simulink model "RobotLocalisation_no_external_mode"  (R2013b)
settings: Solver=FixedStepDiscrete  StartTime=0.0  StopTime=inf  FixedStep=1/30  RelTol=1e-3
PreLoadFcn:
  | force_config
PostLoadFcn:
  | load_scoring_params
values from neighbouring files (symbols this model uses):
  allotedRunTime = 3*60    (= 180)    [load_scoring_params.m]
  startingRadius = 0.1    [load_scoring_params.m]
  startPos = [0.5, 0.5]    [load_scoring_params.m]
  statTimeReq = 2.5    [load_scoring_params.m]
  targetBoundaryRadius = 0.07    [load_scoring_params.m]
undefined symbols (not defined in the file or in its folder): Green, led0, magnitude
libraries: simulink x9, embdlinuxlib x6, visionstatistics x2, visiongeotforms x1
settings Model: ExtModeTrigDuration=100  Creator=omcaree  LastModifiedBy=radams
settings OptimizationCC: InlineParams=on  UseFloatMulNetSlope=on  UseSpecifiedMinMax=on  InlineInvariantSignals=on  EnhancedBackFolding=on  BooleansAsBitfields=on  PassReuseOutputArgsAs=Individual arguments  StateBitsets=on  DataBitsets=on  ZeroExternalMemoryAtStartup=off  ZeroInternalMemoryAtStartup=off  EfficientFloat2IntCast=on  OptimizeModelRefInitCode=on  LifeSpan=1
settings DebuggingCC: SolverPrmCheckMsg=none
settings HardwareCC: ProdLargestAtomicInteger=Long  ProdLargestAtomicFloat=Double  ProdEndianess=LittleEndian  ProdHWDeviceType=ARM Compatible->ARM Cortex
settings RTWCC: SystemTargetFile=realtime.tlc  GenerateMakefile=off  TemplateMakefile=realtime.tmf  Description=Run on Target Hardware  RTWVerbose=off  ProcessScript=realtime_make_rtw_hook  CustomSourceCode="#include \"send_udp.h\""  CustomSource=send_udp.c  IncludeHyperlinkInReport=on  RTWCompilerOptimization=On
settings STFCustomTargetCC: TargetLibSuffix=.a  GenerateSampleERTMain=on  CombineSignalStateStructs=on  SuppressErrorStatus=on  ERTCustomFileBanners=on  SupportNonInlinedSFcns=off  SupportVariableSizeSignals=on  MATLABClassNameForMDSCustomization=Simulink.SoftwareTarget.ERTCustomization  GRTInterface=off  SystemTargetFile=realtime.tlc
settings ERTTargetCC: CodeReplacementLibrary=ANSI_C  GenerateSampleERTMain=on  ParMdlRefBuildCompliant=off  CompOptLevelCompliant=off  ConcurrentExecutionCompliant=off  CombineOutputUpdateFcns=off  CombineSignalStateStructs=on  SuppressErrorStatus=on  ERTFirstTimeCompliant=off  SupportContinuousTime=on  SupportVariableSizeSignals=on  ModelStepFunctionPrototypeControlCompliant=off  CPPClassGenCompliant=off  ExtModeMexArgs='169.254.0.30' 0 17725  InlinedParameterPlacement=NonHierarchical  ERTSrcFileBannerTemplate=realtime_code_template.cgt  ERTHdrFileBannerTemplate=realtime_code_template.cgt  ERTDataSrcFileTemplate=realtime_code_template.cgt  ERTDataHdrFileTemplate=realtime_code_template.cgt  ERTCustomFileTemplate=realtime_file_process.tlc  ConvertIfToSwitch=on  SuppressUnreachableDefaultCases=on

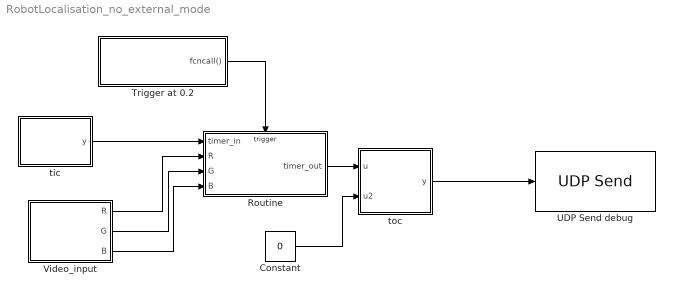
== system RobotLocalisation_no_external_mode ==
  Constant : Constant  Value=0
  Routine : Subsystem  TreatAsAtomicUnit=on
  Trigger at 0.2 : MATLAB Function  TreatAsAtomicUnit=on
  UDP Send debug : embdlinuxlib/UDP Send  remoteURL='169.254.230.213'  remotePort=17728  localURL='255.255.255.255'  localPortSource=Automatically determine  localPort=-1  sampletime=-1  blockPlatform=Raspberry Pi  separateLengthPort=0
  Video_input : Subsystem  TreatAsAtomicUnit=on
  tic : MATLAB Function  TreatAsAtomicUnit=on
  toc : MATLAB Function  TreatAsAtomicUnit=on
  wires:
  Routine/1(timer_out) -> toc/1(u)
  toc/1(y) -> UDP Send debug/1
  tic/1(y) -> Routine/1(timer_in)
  Video_input/1(R) -> Routine/2(R)
  Video_input/2(G) -> Routine/3(G)
  Video_input/3(B) -> Routine/4(B)
  Trigger at 0.2/1(fcncall()) -> Routine/Trigger
  Constant/1 -> toc/2(u2)

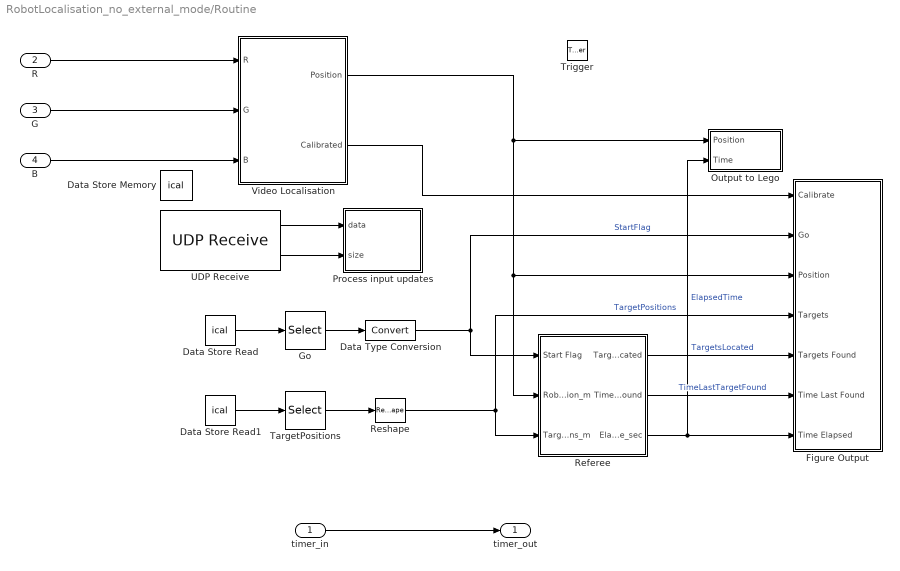
== system RobotLocalisation_no_external_mode/Routine ==
  timer_in : Inport
  R : Inport  Port=2
  G : Inport  Port=3
  B : Inport  Port=4
  Trigger : TriggerPort  TriggerType=function-call  PortDimensions=1
  Data Store Memory : DataStoreMemory  DataStoreName=ical  ReadBeforeWriteMsg=warning  WriteAfterWriteMsg=warning  WriteAfterReadMsg=warning  InitialValue=zeros(22,1)  OutDataTypeStr=double
  Data Store Read : DataStoreRead  DataStoreName=ical
  Data Store Read1 : DataStoreRead  DataStoreName=ical
  Data Type Conversion : DataTypeConversion
  Figure Output : Subsystem
  Go : Selector  InputPortWidth=22  IndexOptions=Index vector (dialog)  Indices=1  OutputSizes=1
  Output to Lego : Subsystem
  Process input updates : MATLAB Function  TreatAsAtomicUnit=on
  Referee : Subsystem
      mask Display: image(imread('referee.png'))
  Reshape : Reshape  OutputDimensionality=Customize  OutputDimensions=[9 2]
  TargetPositions : Selector  InputPortWidth=22  IndexOptions=Index vector (dialog)  Indices=[2:19]  OutputSizes=1
  UDP Receive : embdlinuxlib/UDP Receive  localURL='0.0.0.0'  localPort=17727  remoteURL='0.0.0.0'  remotePort=-1  recvBufferSize=8192  signalDatatype=uint8  dims=176  isVarSize=off  showBlockingTime=off  blockingTime=0  sampletime=-1  blockPlatform=Raspberry Pi
  Video Localisation : Subsystem
  timer_out : Outport
  wires:
  Data Type Conversion/1 -> Referee/1(Start Flag), Figure Output/2(Go)  "StartFlag"
  Referee/1(Targets Located) -> Figure Output/5(Targets Found)  "TargetsLocated"
  Reshape/1 -> Referee/3(Target Positions_m), Figure Output/4(Targets)  "TargetPositions"
  Video Localisation/1(Position) -> Referee/2(Robot Position_m), Figure Output/3(Position), Output to Lego/1(Position)
  Video Localisation/2(Calibrated) -> Figure Output/1(Calibrate)
  Referee/2(Time Last Target Found) -> Figure Output/6(Time Last Found)  "TimeLastTargetFound"
  Referee/3(Elapsed Time_sec) -> Output to Lego/2(Time), Figure Output/7(Time Elapsed)  "ElapsedTime"
  UDP Receive/1 -> Process input updates/1(data)
  UDP Receive/2 -> Process input updates/2(size)
  Data Store Read/1 -> Go/1
  Go/1 -> Data Type Conversion/1
  TargetPositions/1 -> Reshape/1
  Data Store Read1/1 -> TargetPositions/1
  timer_in/1 -> timer_out/1
  R/1 -> Video Localisation/1(R)
  G/1 -> Video Localisation/2(G)
  B/1 -> Video Localisation/3(B)

== system RobotLocalisation_no_external_mode/Video_input ==
  V4L2 Video Capture : embdlinuxlib/V4L2 Video Capture  m_devName='/dev/video0'  roi=[0, 0, 640, 480]  imSizeSelection=320x240  imSize=[640, 480]  pixelFormat=RGB  pixelOrder=Planar  sampleTime=1/30  simOutput=Colorbars  blockPlatform=Raspberry Pi
  R : Outport
  G : Outport  Port=2
  B : Outport  Port=3
  wires:
  V4L2 Video Capture/3 -> B/1
  V4L2 Video Capture/2 -> G/1
  V4L2 Video Capture/1 -> R/1

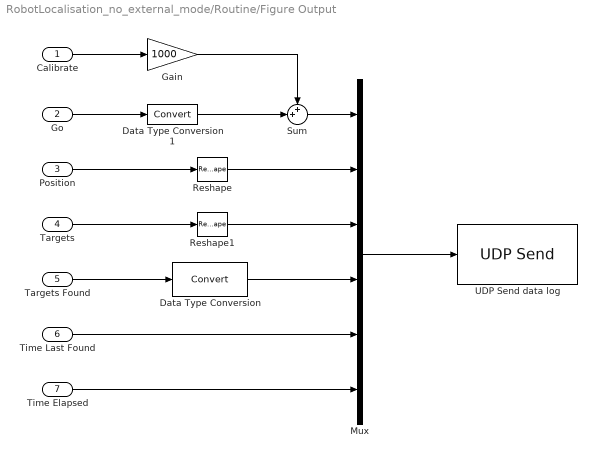
== system RobotLocalisation_no_external_mode/Routine/Figure Output ==
  Calibrate : Inport
  Go : Inport  Port=2
  Position : Inport  Port=3
  Targets : Inport  Port=4
  Targets Found : Inport  Port=5
  Time Last Found : Inport  Port=6
  Time Elapsed : Inport  Port=7
  Data Type Conversion : DataTypeConversion
  Data Type Conversion1 : DataTypeConversion
  Gain : Gain  Gain=1000  OutDataTypeStr=double
  Mux : Mux  Inputs=6
  Reshape : Reshape
  Reshape1 : Reshape
  Sum : Sum  Inputs=++|
  UDP Send data log : embdlinuxlib/UDP Send  remoteURL='169.254.230.213'  remotePort=17726  localURL='255.255.255.255'  localPortSource=Automatically determine  localPort=-1  sampletime=-1  blockPlatform=Raspberry Pi  separateLengthPort=0
  wires:
  Targets/1 -> Reshape1/1
  Targets Found/1 -> Data Type Conversion/1
  Time Last Found/1 -> Mux/5
  Time Elapsed/1 -> Mux/6
  Mux/1 -> UDP Send data log/1
  Position/1 -> Reshape/1
  Data Type Conversion/1 -> Mux/4
  Reshape/1 -> Mux/2
  Reshape1/1 -> Mux/3
  Calibrate/1 -> Gain/1
  Sum/1 -> Mux/1
  Go/1 -> Data Type Conversion1/1
  Gain/1 -> Sum/1
  Data Type Conversion1/1 -> Sum/2

== system RobotLocalisation_no_external_mode/Routine/Output to Lego ==
  Position : Inport
  Time : Inport  Port=2
  Data Type Conversion1 : DataTypeConversion  OutDataTypeStr=int32
  Demux1 : Demux  Outputs=2
  Gain3 : Gain  Gain=10  ParamDataTypeStr=uint8
  Gain4 : Gain  Gain=100  ParamDataTypeStr=uint8
  Gain5 : Gain  Gain=100  ParamDataTypeStr=uint8
  Mux1 : Mux  Inputs=3
  UDP Send2 : embdlinuxlib/UDP Send  remoteURL='127.0.0.1'  remotePort=32000  localURL='255.255.255.255'  localPortSource=Automatically determine  localPort=-1  sampletime=-1  blockPlatform=Raspberry Pi  separateLengthPort=0
  wires:
  Position/1 -> Demux1/1
  Time/1 -> Gain3/1
  Mux1/1 -> Data Type Conversion1/1
  Data Type Conversion1/1 -> UDP Send2/1
  Demux1/1 -> Gain4/1
  Demux1/2 -> Gain5/1
  Gain4/1 -> Mux1/2
  Gain5/1 -> Mux1/3
  Gain3/1 -> Mux1/1

== system RobotLocalisation_no_external_mode/Routine/Referee ==
  Start Flag : Inport  OutDataTypeStr=boolean
  Robot Position_m : Inport  Port=2
  Target Positions_m : Inport  Port=3
  Chart (MATLAB) : Stateflow chart  TreatAsAtomicUnit=on
  Reshape : Reshape  OutputDimensionality=Row vector (2-D)
  Targets Located : Outport
  Time Last Target Found : Outport  Port=2  PortDimensions=1
  Elapsed Time_sec : Outport  Port=3  PortDimensions=1
  wires:
  Chart (MATLAB)/1(timeLastTargetFound) -> Time Last Target Found/1
  Chart (MATLAB)/3(targetsFound) -> Targets Located/1
  Robot Position_m/1 -> Reshape/1
  Start Flag/1 -> Chart (MATLAB)/2(StartFlag)
  Reshape/1 -> Chart (MATLAB)/1(robotPosition)
  Target Positions_m/1 -> Chart (MATLAB)/3(targetPositions)
  Chart (MATLAB)/2(elapsedTime) -> Elapsed Time_sec/1

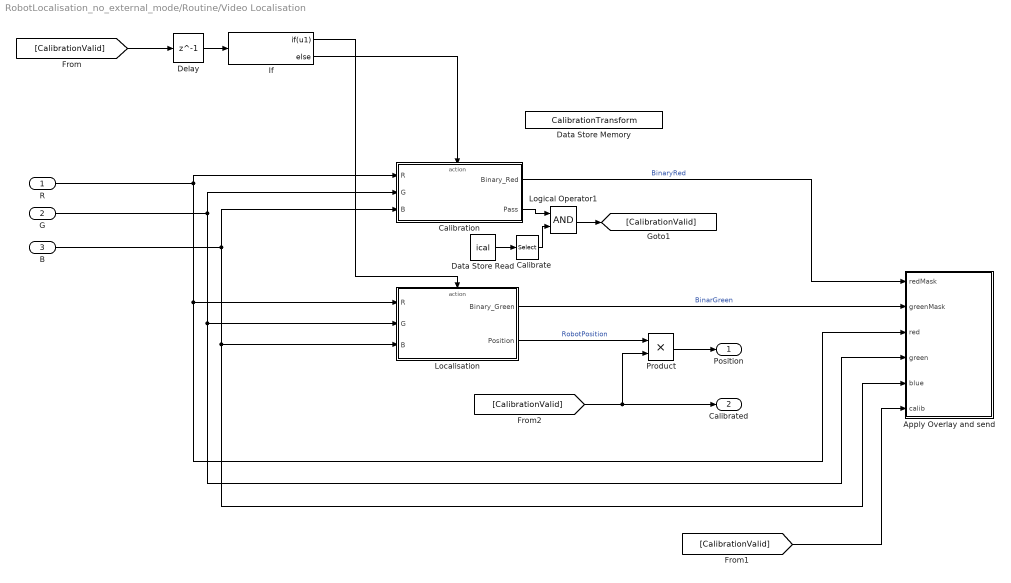
== system RobotLocalisation_no_external_mode/Routine/Video Localisation ==
  R : Inport
  G : Inport  Port=2
  B : Inport  Port=3
  Apply Overlay and send : MATLAB Function
  Calibrate : Selector  InputPortWidth=22  IndexOptions=Index vector (dialog)  Indices=22  OutputSizes=1
  Calibration : Subsystem  TreatAsAtomicUnit=on
      settings: RTWSystemCode=Inline
  Data Store Memory : DataStoreMemory  DataStoreName=CalibrationTransform  ReadBeforeWriteMsg=warning  WriteAfterWriteMsg=warning  WriteAfterReadMsg=warning  InitialValue=[1 0 0; 0 1 0; 0 0 1]  VectorParams1D=off  Dimensions=[3 3]
  Data Store Read : DataStoreRead  DataStoreName=ical
  Delay : Delay  DelayLength=1  InitialCondition=0
  If : If  IfExpression=u1
  Localisation : Subsystem  TreatAsAtomicUnit=on
      settings: RTWSystemCode=Inline
  Logical Operator1 : Logic  AllPortsSameDT=off  OutDataTypeStr=boolean
  Product : Product  OutDataTypeStr=double
  Position : Outport
  Calibrated : Outport  Port=2
  wires:
  Delay/1 -> If/1
  [CalibrationValid] -> Delay/1
  Localisation/2(Position) -> Product/1  "RobotPosition"
  Product/1 -> Position/1
  Data Store Read/1 -> Calibrate/1
  Calibration/2(Pass) -> Logical Operator1/1
  Calibrate/1 -> Logical Operator1/2
  Logical Operator1/1 -> [CalibrationValid]
  [CalibrationValid] -> Product/2, Calibrated/1
  Calibration/1(Binary_Red) -> Apply Overlay and send/1(redMask)  "BinaryRed"
  Localisation/1(Binary_Green) -> Apply Overlay and send/2(greenMask)  "BinarGreen"
  R/1 -> Calibration/1(R), Apply Overlay and send/3(red), Localisation/1(R)
  G/1 -> Apply Overlay and send/4(green), Localisation/2(G), Calibration/2(G)
  B/1 -> Calibration/3(B), Apply Overlay and send/5(blue), Localisation/3(B)
  If/2 -> Calibration/Action
  If/1 -> Localisation/Action
  [CalibrationValid] -> Apply Overlay and send/6(calib)

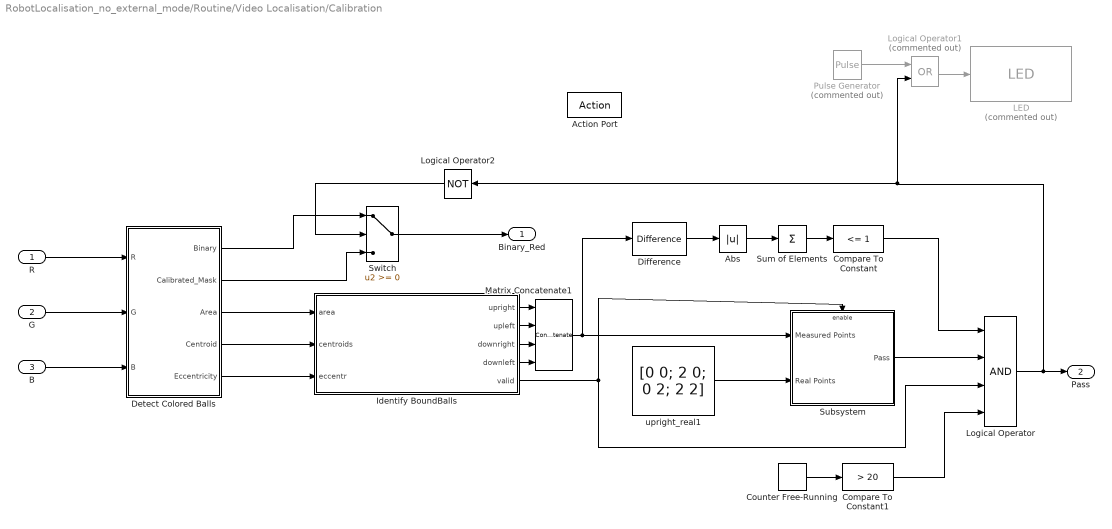
== system RobotLocalisation_no_external_mode/Routine/Video Localisation/Calibration ==
  R : Inport
  G : Inport  Port=2
  B : Inport  Port=3
  Action Port : ActionPort  ActionType=else
  Abs : Abs
  Compare To Constant : simulink/Logic and Bit Operations/Compare To Constant  relop=<=  const=1  OutDataTypeStr=boolean
  Compare To Constant1 : simulink/Logic and Bit Operations/Compare To Constant  relop=>  const=20  OutDataTypeStr=boolean
  Counter Free-Running : simulink/Sources/Counter Free-Running  NumBits=16  tsamp=-1
  Detect Colored Balls : Subsystem
  Difference : simulink/Discrete/Difference  ICPrevInput=0.0  InputProcessing=Inherited  OutMin=[]  OutMax=[]  OutDataType=fixdt(1, 16)  OutScaling=2^-10  DoSatur=off
  Identify BoundBalls : MATLAB Function  TreatAsAtomicUnit=on
  LED : embdlinuxlib/LED  Commented=on  board=Model B Rev2  led=led0 (Green)  blockPlatform=Raspberry Pi
  Logical Operator : Logic  Inputs=4  AllPortsSameDT=off  OutDataTypeStr=boolean
  Logical Operator1 : Logic  Commented=on  Operator=OR  AllPortsSameDT=off  OutDataTypeStr=boolean
  Logical Operator2 : Logic  Operator=NOT  AllPortsSameDT=off  OutDataTypeStr=boolean
  Matrix Concatenate1 : Concatenate  NumInputs=4  Mode=Multidimensional array
  Pulse Generator : DiscretePulseGenerator  Commented=on  PulseType=Time based  Period=0.4  PulseWidth=50
  Subsystem : Subsystem
  Sum of Elements : Sum  Inputs=+
  Switch : Switch
  upright_real1 : Constant  Value=[0 0; 2 0; 0 2; 2 2]  VectorParams1D=off
  Binary_Red : Outport
  Pass : Outport  Port=2
  wires:
  Identify BoundBalls/2(upleft) -> Matrix Concatenate1/2
  Identify BoundBalls/3(downright) -> Matrix Concatenate1/3
  Identify BoundBalls/4(downleft) -> Matrix Concatenate1/4
  Identify BoundBalls/1(upright) -> Matrix Concatenate1/1
  Matrix Concatenate1/1 -> Difference/1, Subsystem/1(Measured Points)
  Identify BoundBalls/5(valid) -> Logical Operator/3, Subsystem/Enable
  Difference/1 -> Abs/1
  Sum of Elements/1 -> Compare To Constant/1
  Abs/1 -> Sum of Elements/1
  Compare To Constant/1 -> Logical Operator/1
  R/1 -> Detect Colored Balls/1(R)
  G/1 -> Detect Colored Balls/2(G)
  B/1 -> Detect Colored Balls/3(B)
  Detect Colored Balls/3(Area) -> Identify BoundBalls/1(area)
  Detect Colored Balls/4(Centroid) -> Identify BoundBalls/2(centroids)
  Detect Colored Balls/5(Eccentricity) -> Identify BoundBalls/3(eccentr)
  Subsystem/1(Pass) -> Logical Operator/2
  Logical Operator/1 -> Pass/1, Logical Operator1/2, Logical Operator2/1
  Pulse Generator/1 -> Logical Operator1/1
  Logical Operator1/1 -> LED/1
  Counter Free-Running/1 -> Compare To Constant1/1
  Compare To Constant1/1 -> Logical Operator/4
  upright_real1/1 -> Subsystem/2(Real Points)
  Detect Colored Balls/1(Binary) -> Switch/1
  Detect Colored Balls/2(Calibrated_Mask) -> Switch/3
  Switch/1 -> Binary_Red/1
  Logical Operator2/1 -> Switch/2

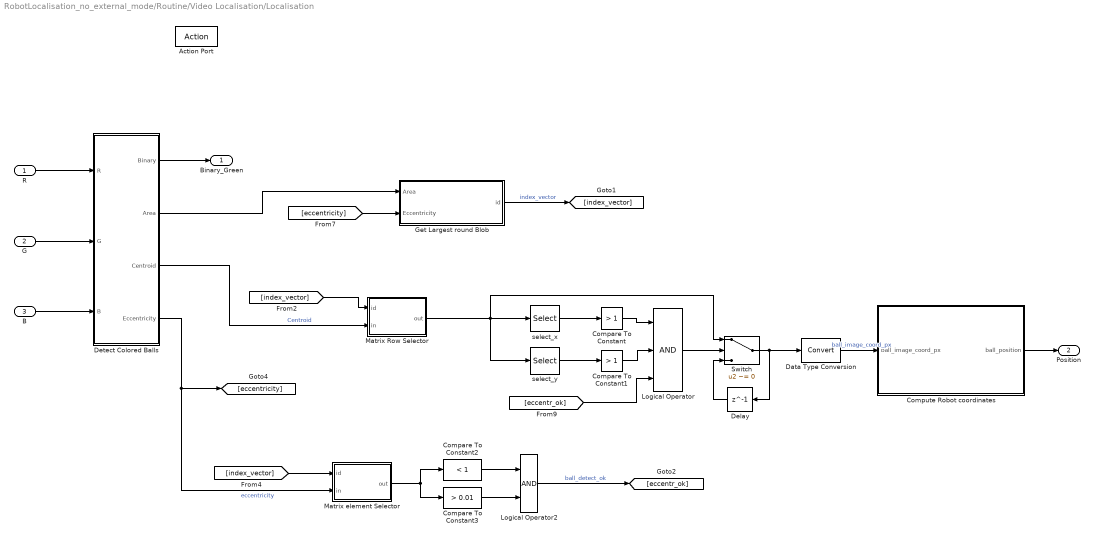
== system RobotLocalisation_no_external_mode/Routine/Video Localisation/Localisation ==
  R : Inport
  G : Inport  Port=2
  B : Inport  Port=3
  Action Port : ActionPort  ActionType=then
  Compare To Constant : simulink/Logic and Bit Operations/Compare To Constant  relop=>  const=1  OutDataTypeStr=boolean
  Compare To Constant1 : simulink/Logic and Bit Operations/Compare To Constant  relop=>  const=1  OutDataTypeStr=boolean
  Compare To Constant2 : simulink/Logic and Bit Operations/Compare To Constant  relop=<  const=1  OutDataTypeStr=boolean
  Compare To Constant3 : simulink/Logic and Bit Operations/Compare To Constant  relop=>  const=0.01  OutDataTypeStr=boolean
  Compute Robot coordinates : Subsystem
  Data Type Conversion : DataTypeConversion
  Delay : Delay  DelayLength=1  InitialCondition=320/2
  Detect Colored Balls : Subsystem
  Get Largest round Blob : MATLAB Function  TreatAsAtomicUnit=on
  Logical Operator : Logic  Inputs=3  AllPortsSameDT=off  OutDataTypeStr=boolean
  Logical Operator2 : Logic  AllPortsSameDT=off  OutDataTypeStr=boolean
  Matrix Row Selector : MATLAB Function  TreatAsAtomicUnit=on
  Matrix element Selector : MATLAB Function  TreatAsAtomicUnit=on
  Switch : Switch  Criteria=u2 ~= 0
  select_x : Selector  InputPortWidth=2  IndexOptions=Index vector (dialog)  Indices=[1 ]  OutputSizes=1
  select_y : Selector  InputPortWidth=2  IndexOptions=Index vector (dialog)  Indices=2  OutputSizes=1
  Binary_Green : Outport
  Position : Outport  Port=2
  wires:
  B/1 -> Detect Colored Balls/3(B)
  G/1 -> Detect Colored Balls/2(G)
  R/1 -> Detect Colored Balls/1(R)
  Detect Colored Balls/2(Area) -> Get Largest round Blob/1(Area)
  Switch/1 -> Data Type Conversion/1, Delay/1
  Delay/1 -> Switch/3
  select_x/1 -> Compare To Constant/1
  Compare To Constant/1 -> Logical Operator/1
  Logical Operator/1 -> Switch/2
  Get Largest round Blob/1(id) -> [index_vector]  "index_vector"
  Compare To Constant2/1 -> Logical Operator2/1
  Detect Colored Balls/4(Eccentricity) -> Matrix element Selector/2(in), [eccentricity]  "eccentricity"
  [index_vector] -> Matrix element Selector/1(id)
  Detect Colored Balls/3(Centroid) -> Matrix Row Selector/2(in)  "Centroid"
  [index_vector] -> Matrix Row Selector/1(id)
  Matrix Row Selector/1(out) -> select_y/1, select_x/1, Switch/1
  Matrix element Selector/1(out) -> Compare To Constant2/1, Compare To Constant3/1
  Compare To Constant3/1 -> Logical Operator2/2
  Logical Operator2/1 -> [eccentr_ok]  "ball_detect_ok"
  [eccentricity] -> Get Largest round Blob/2(Eccentricity)
  Data Type Conversion/1 -> Compute Robot coordinates/1(ball_image_coord_px)  "ball_image_coord_px"
  select_y/1 -> Compare To Constant1/1
  Compare To Constant1/1 -> Logical Operator/2
  [eccentr_ok] -> Logical Operator/3
  Compute Robot coordinates/1(ball_position) -> Position/1
  Detect Colored Balls/1(Binary) -> Binary_Green/1

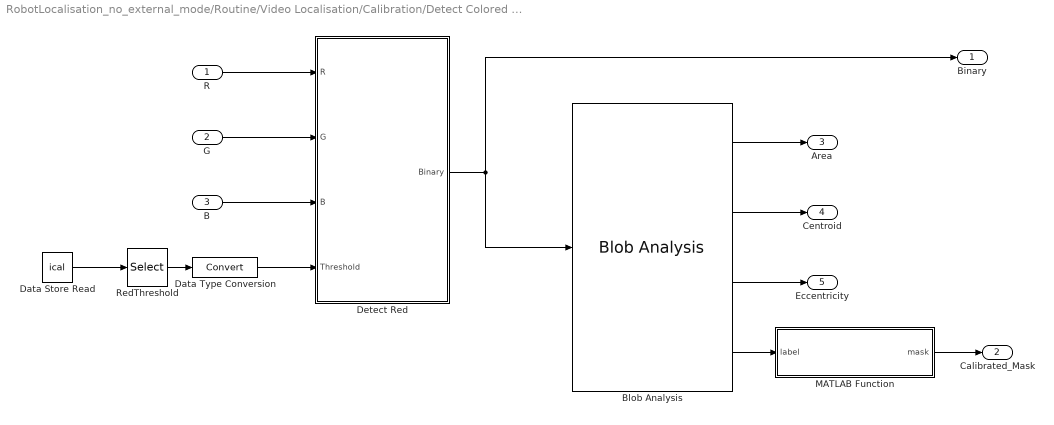
== system RobotLocalisation_no_external_mode/Routine/Video Localisation/Calibration/Detect Colored Balls ==
  R : Inport
  G : Inport  Port=2
  B : Inport  Port=3
  Blob Analysis : visionstatistics/Blob Analysis  Tag=vipblks_row_conv  area=on  centroid=on  bBox=off  majorAxis=off  minorAxis=off  angle=off  eccentricity=on  equivDiameterSq=off  extent=off  perimeter=off  maxBlobs=4  warnIfNumBlobsExceeded=on  isCount=off  useMinArea=on  minArea=10  useMaxArea=off  maxArea=15000  excludeBorderBlob=on  outDT=double  isOutVarDim=off  isFill=on  fillValues=0  conn=4  isLabel=on  outputMode=Binary point scaling  outputWordLength=32  outputFracLength=16  firstCoeffMode=Binary point scaling  firstCoeffWordLength=16  firstCoeffFracLength=14  secondCoeffMode=Binary point scaling  secondCoeffWordLength=32  secondCoeffFracLength=16  accumMode=Binary point scaling  accumWordLength=32  accumFracLength=0  prodOutputMode=Binary point scaling  prodOutputWordLength=32  prodOutputFracLength=16  roundingMode=Floor  overflowMode=off
  Data Store Read : DataStoreRead  DataStoreName=ical
  Data Type Conversion : DataTypeConversion
  Detect Red : Subsystem
  MATLAB Function : MATLAB Function  TreatAsAtomicUnit=on
  RedThreshold : Selector  InputPortWidth=22  IndexOptions=Index vector (dialog)  Indices=20  OutputSizes=1
  Binary : Outport
  Calibrated_Mask : Outport  Port=2
  Area : Outport  Port=3
  Centroid : Outport  Port=4
  Eccentricity : Outport  Port=5
  wires:
  G/1 -> Detect Red/2(G)
  R/1 -> Detect Red/1(R)
  B/1 -> Detect Red/3(B)
  Detect Red/1(Binary) -> Binary/1, Blob Analysis/1
  Blob Analysis/2 -> Centroid/1
  Blob Analysis/1 -> Area/1
  Blob Analysis/3 -> Eccentricity/1
  Data Store Read/1 -> RedThreshold/1
  RedThreshold/1 -> Data Type Conversion/1
  Data Type Conversion/1 -> Detect Red/4(Threshold)
  Blob Analysis/4 -> MATLAB Function/1(label)
  MATLAB Function/1(mask) -> Calibrated_Mask/1

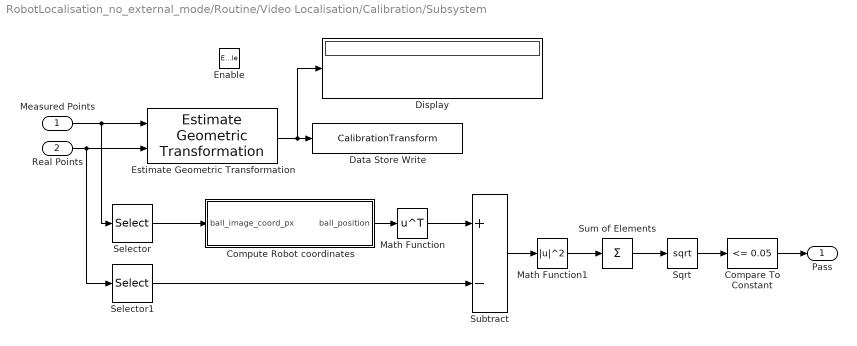
== system RobotLocalisation_no_external_mode/Routine/Video Localisation/Calibration/Subsystem ==
  Measured Points : Inport
  Real Points : Inport  Port=2
  Enable : EnablePort
  Compare To Constant : simulink/Logic and Bit Operations/Compare To Constant  relop=<=  const=0.05  OutDataTypeStr=boolean
  Compute Robot coordinates : Subsystem
  Data Store Write : DataStoreWrite  DataStoreName=CalibrationTransform
  Display : Display
  Estimate Geometric Transformation : visiongeotforms/Estimate Geometric Transformation  tformType=Projective  isRandomSampling=on  algMethod=Random Sample Consensus (RANSAC)  numMethod=Specified value  isStopSampling=off  percentStop=75  distanceAlg=2.5  distanceGeo=2.5  sampleNum=500  maxSampleNum=1000  desiredConfidence=99  isRefineTForm=off  isOutputInlier=off  outDT4IntInput=Obsolete10a  outDT4IntInputActive=Single  isVarSizeAllowed=on  isReleaseMode=on
  Math Function1 : Math  Operator=magnitude^2  SaturateOnIntegerOverflow=on
  Math Function : Math  Operator=transpose  SaturateOnIntegerOverflow=on
  Selector : Selector  NumberOfDimensions=2  InputPortWidth=3  IndexOptions=Index vector (dialog),Select all  Indices=1,1  OutputSizes=1,1
  Selector1 : Selector  NumberOfDimensions=2  InputPortWidth=3  IndexOptions=Index vector (dialog),Select all  Indices=1,1  OutputSizes=1,1
  Sqrt : Sqrt  SaturateOnIntegerOverflow=on
  Subtract : Sum  Inputs=+-
  Sum of Elements : Sum  Inputs=+
  Pass : Outport
  wires:
  Estimate Geometric Transformation/1 -> Display/1, Data Store Write/1
  Real Points/1 -> Selector1/1, Estimate Geometric Transformation/2
  Measured Points/1 -> Selector/1, Estimate Geometric Transformation/1
  Selector/1 -> Compute Robot coordinates/1(ball_image_coord_px)
  Compute Robot coordinates/1(ball_position) -> Math Function/1
  Subtract/1 -> Math Function1/1
  Sqrt/1 -> Compare To Constant/1
  Compare To Constant/1 -> Pass/1
  Math Function/1 -> Subtract/1
  Math Function1/1 -> Sum of Elements/1
  Sum of Elements/1 -> Sqrt/1
  Selector1/1 -> Subtract/2

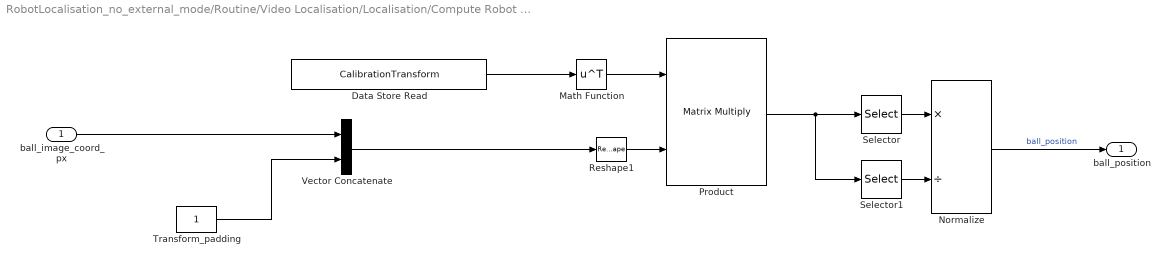
== system RobotLocalisation_no_external_mode/Routine/Video Localisation/Localisation/Compute Robot coordinates ==
  ball_image_coord_px : Inport
  Data Store Read : DataStoreRead  DataStoreName=CalibrationTransform
  Math Function : Math  Operator=transpose  SaturateOnIntegerOverflow=on
  Normalize : Product  Inputs=*/  RndMeth=Zero
  Product : Product  Multiplication=Matrix(*)  RndMeth=Zero
  Reshape1 : Reshape  OutputDimensionality=Column vector (2-D)  OutputDimensions=[2,1]
  Selector : Selector  InputPortWidth=3  IndexOptions=Index vector (dialog)  Indices=[1 2]  OutputSizes=1
  Selector1 : Selector  InputPortWidth=3  IndexOptions=Index vector (dialog)  Indices=[3]  OutputSizes=1
  Transform_padding : Constant
  Vector Concatenate : Concatenate
  ball_position : Outport
  wires:
  ball_image_coord_px/1 -> Vector Concatenate/1
  Transform_padding/1 -> Vector Concatenate/2
  Data Store Read/1 -> Math Function/1
  Vector Concatenate/1 -> Reshape1/1
  Math Function/1 -> Product/1
  Reshape1/1 -> Product/2
  Product/1 -> Selector1/1, Selector/1
  Selector/1 -> Normalize/1
  Selector1/1 -> Normalize/2
  Normalize/1 -> ball_position/1  "ball_position"

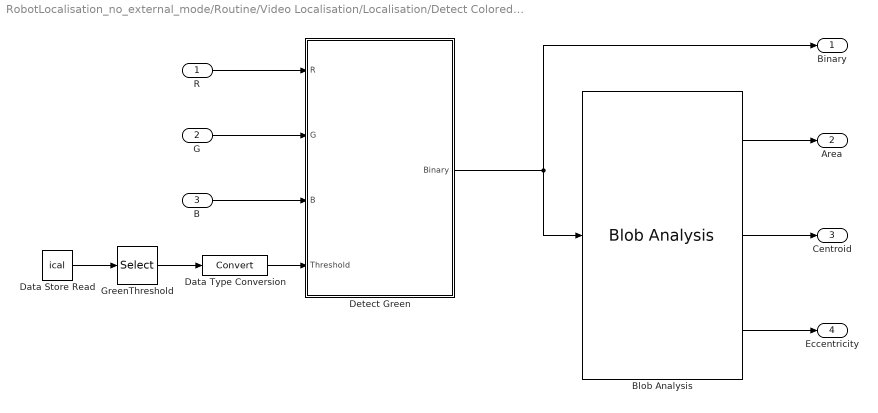
== system RobotLocalisation_no_external_mode/Routine/Video Localisation/Localisation/Detect Colored Balls ==
  R : Inport
  G : Inport  Port=2
  B : Inport  Port=3
  Blob Analysis : visionstatistics/Blob Analysis  Tag=vipblks_row_conv  area=on  centroid=on  bBox=off  majorAxis=off  minorAxis=off  angle=off  eccentricity=on  equivDiameterSq=off  extent=off  perimeter=off  maxBlobs=10  warnIfNumBlobsExceeded=on  isCount=off  useMinArea=on  minArea=10  useMaxArea=off  maxArea=15000  excludeBorderBlob=on  outDT=double  isOutVarDim=off  isFill=on  fillValues=0  conn=4  isLabel=off  outputMode=Binary point scaling  outputWordLength=32  outputFracLength=16  firstCoeffMode=Binary point scaling  firstCoeffWordLength=16  firstCoeffFracLength=14  secondCoeffMode=Binary point scaling  secondCoeffWordLength=32  secondCoeffFracLength=16  accumMode=Binary point scaling  accumWordLength=32  accumFracLength=0  prodOutputMode=Binary point scaling  prodOutputWordLength=32  prodOutputFracLength=16  roundingMode=Floor  overflowMode=off
  Data Store Read : DataStoreRead  DataStoreName=ical
  Data Type Conversion : DataTypeConversion
  Detect Green : Subsystem
  GreenThreshold : Selector  InputPortWidth=22  IndexOptions=Index vector (dialog)  Indices=21  OutputSizes=1
  Binary : Outport
  Area : Outport  Port=2
  Centroid : Outport  Port=3
  Eccentricity : Outport  Port=4
  wires:
  G/1 -> Detect Green/2(G)
  R/1 -> Detect Green/1(R)
  B/1 -> Detect Green/3(B)
  Detect Green/1(Binary) -> Binary/1, Blob Analysis/1
  GreenThreshold/1 -> Data Type Conversion/1
  Blob Analysis/2 -> Centroid/1
  Blob Analysis/1 -> Area/1
  Blob Analysis/3 -> Eccentricity/1
  Data Store Read/1 -> GreenThreshold/1
  Data Type Conversion/1 -> Detect Green/4(Threshold)

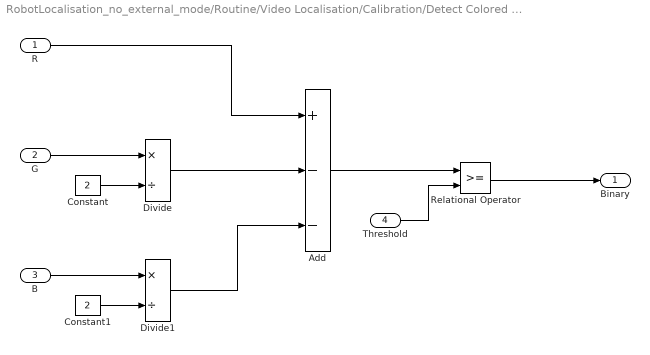
== system RobotLocalisation_no_external_mode/Routine/Video Localisation/Calibration/Detect Colored Balls/Detect Red ==
  R : Inport
  G : Inport  Port=2
  B : Inport  Port=3
  Threshold : Inport  Port=4
  Add : Sum  Inputs=+--  OutDataTypeStr=uint8  SaturateOnIntegerOverflow=on
  Constant : Constant  Value=2  OutDataTypeStr=uint8
  Constant1 : Constant  Value=2  OutDataTypeStr=uint8
  Divide : Product  Inputs=*/
  Divide1 : Product  Inputs=*/
  Relational Operator : RelationalOperator  OutDataTypeStr=boolean
  Binary : Outport
  wires:
  G/1 -> Divide/1
  B/1 -> Divide1/1
  Threshold/1 -> Relational Operator/2
  Relational Operator/1 -> Binary/1
  Divide/1 -> Add/2
  Divide1/1 -> Add/3
  Add/1 -> Relational Operator/1
  Constant/1 -> Divide/2
  R/1 -> Add/1
  Constant1/1 -> Divide1/2

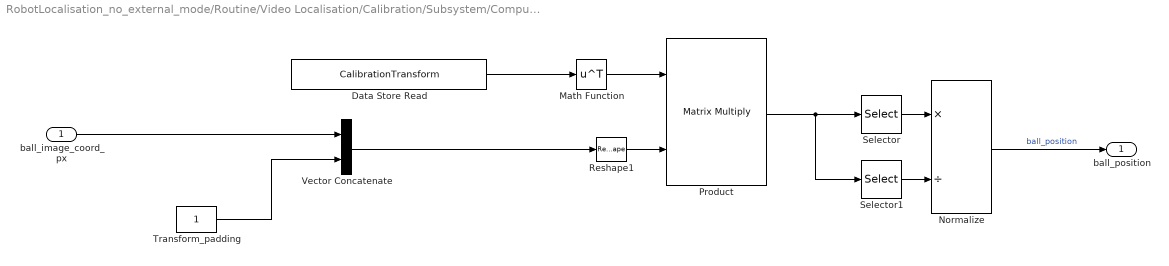
== system RobotLocalisation_no_external_mode/Routine/Video Localisation/Calibration/Subsystem/Compute Robot coordinates ==
  ball_image_coord_px : Inport
  Data Store Read : DataStoreRead  DataStoreName=CalibrationTransform
  Math Function : Math  Operator=transpose  SaturateOnIntegerOverflow=on
  Normalize : Product  Inputs=*/  RndMeth=Zero
  Product : Product  Multiplication=Matrix(*)  RndMeth=Zero
  Reshape1 : Reshape  OutputDimensionality=Column vector (2-D)  OutputDimensions=[2,1]
  Selector : Selector  InputPortWidth=3  IndexOptions=Index vector (dialog)  Indices=[1 2]  OutputSizes=1
  Selector1 : Selector  InputPortWidth=3  IndexOptions=Index vector (dialog)  Indices=[3]  OutputSizes=1
  Transform_padding : Constant
  Vector Concatenate : Concatenate
  ball_position : Outport
  wires:
  ball_image_coord_px/1 -> Vector Concatenate/1
  Transform_padding/1 -> Vector Concatenate/2
  Data Store Read/1 -> Math Function/1
  Vector Concatenate/1 -> Reshape1/1
  Math Function/1 -> Product/1
  Reshape1/1 -> Product/2
  Product/1 -> Selector1/1, Selector/1
  Selector/1 -> Normalize/1
  Selector1/1 -> Normalize/2
  Normalize/1 -> ball_position/1  "ball_position"

== system RobotLocalisation_no_external_mode/Routine/Video Localisation/Localisation/Detect Colored Balls/Detect Green ==
  R : Inport
  G : Inport  Port=2
  B : Inport  Port=3
  Threshold : Inport  Port=4
  Add : Sum  Inputs=-+-  OutDataTypeStr=uint8  SaturateOnIntegerOverflow=on
  Constant : Constant  Value=2  OutDataTypeStr=uint8
  Constant1 : Constant  Value=2  OutDataTypeStr=uint8
  Divide : Product  Inputs=*/
  Divide1 : Product  Inputs=*/
  Relational Operator : RelationalOperator  OutDataTypeStr=boolean
  Binary : Outport
  wires:
  Threshold/1 -> Relational Operator/2
  Relational Operator/1 -> Binary/1
  G/1 -> Add/2
  Add/1 -> Relational Operator/1
  R/1 -> Divide/1
  Divide/1 -> Add/1
  B/1 -> Divide1/1
  Divide1/1 -> Add/3
  Constant/1 -> Divide/2
  Constant1/1 -> Divide1/2

== stateflow chart RobotLocalisation_no_external_mode/Routine/Referee/Chart (MATLAB) ==
  state Standby
    entry:
    numTargets = size(targetPositions,1);
    targetsFound = false(size(targetPositions,1),1);
    timeLastTargetFound = 0;
    elapsedTime = 0;
    numTargetsFound = 0;
  state Running
    entry: startTiming;
    during:
    elapsedTime = getTiming;
    [nearLocation, currentTarget] = testIfNearLocation(robotPosition, targetPositions, targetBoundaryRadius);
    state NearLocation
      entry: snapshotTime = elapsedTime
    state Roaming
    Roaming -> NearLocation : [nearLocation == true]
    (default) -> Roaming
    NearLocation -> Roaming [order 2] : [nearLocation == false]
    NearLocation -> (junction 43) [order 1] : [(elapsedTime - snapshotTime) > statTimeReq]
    (junction 44) -> Roaming
    (junction 43) -> (junction 44) : {[targetsFound, timeLastTargetFound] = ...
        | updateTargetsFound(targetsFound, currentTarget, timeLastTargetFound,elapsedTime);
        | numTargetsFound = sum(targetsFound);}
  state Finished
  Finished -> Standby : [StartFlag == false]
  (default) -> Standby
  Standby -> Running : [StartFlag == true &&...
      | distancefrom(robotPosition, startPos) < startingRadius ]
  Running -> Standby [order 2] : [StartFlag == false]
  Running -> Finished [order 1] : [numTargetsFound == numTargets ||...
      |  elapsedTime >= allotedRunTime-sqrt(eps)]
  data: et function_output; tfound_in function_input; currentT function_input; tfound_out function_output; lastTime_in function_input; lastTime_out function_output; time function_input; robotPos function_input; targetPos function_input; proximityVal function_input; nearLoc function_output; currentLoc function_output; pos function_input; x0 function_input; d function_output; startPos parameter; allotedRunTime parameter; statTimeReq parameter; startingRadius parameter; robotPosition input; targetBoundaryRadius parameter; StartFlag input; targetPositions input; timeLastTargetFound output; nearLocation local; numTargetsFound local; elapsedTime output; numTargets local; currentTarget local; targetsFound output; snapshotTime local
  function startTiming:
    | function startTiming
    |  
    | if strcmp(coder.target,'rtw')
    |     coder.ceval('tic',int32(2));
    | end
  function et = getTiming:
    | function et = getTiming
    | 
    | lt = 0;
    | 
    | if strcmp(coder.target,'rtw')
    |     coder.ceval('toc',coder.wref(lt),int32(2));
    | end
    | 
    | et = lt;
  function [tfound_out, lastTime_out] = updateTargetsFound(tfound_in, currentT, lastTime_in, time):
    | function [tfound_out, lastTime_out] = updateTargetsFound(tfound_in, currentT, lastTime_in, time)
    | 
    | if any(tfound_in & currentT) %is this an existing target
    |     lastTime_out = lastTime_in;
    | else
    |     lastTime_out = time;
    | end
    | 
    | tfound_out = tfound_in | currentT; %update list of found targets
  function [nearLoc, currentLoc] = testIfNearLocation(robotPos, targetPos, proximityVal):
    | function [nearLoc, currentLoc] = testIfNearLocation(robotPos, targetPos, proximityVal)
    | %#codegen
    | delta = bsxfun(@minus, targetPos, robotPos);
    | dist = sum(delta.^2,2);
    | 
    | currentLoc = dist <= proximityVal^2;
    | nearLoc = any(currentLoc);
  function d = distancefrom(pos,x0):
    | function d = distancefrom(pos,x0)
    | d = sqrt(sum((pos-x0).^2));

== matlab function RobotLocalisation_no_external_mode/Routine/Video Localisation/Calibration/Detect Colored Balls/MATLAB Function ==
  data: label input; mask output
function mask = rescale_mask(label)
%#codegen

mask = logical(min(uint8(label),uint8(1)));

== matlab function RobotLocalisation_no_external_mode/Routine/Video Localisation/Calibration/Identify BoundBalls ==
  data: area input; centroids input; upright output size=[1 2]; upleft output size=[1 2]; downright output size=[1 2]; downleft output size=[1 2]; eccentr input; valid output
function [upright, upleft, downright, downleft, valid] = identitfyBoundBall(area,centroids,eccentr)
% This block supports the Embedded MATLAB subset.
% See the help menu for details. 


%% Select and Sort candidate markers
% Pick the biggest and roundest blobs


criteria = double(area)+1./(1+10*eccentr);
[~,sorted_idx] = sort(criteria,'descend');

candidates_idx = sorted_idx(1:4);
candidates = centroids(candidates_idx,:);

% Find upper and lower round blobs
[~,upper_idx] = sort(candidates(:,2));

candidates_up = candidates(upper_idx(1:2),:);
candidates_down = candidates(upper_idx(3:4),:);

[~,left_idx] = sort(candidates_up(:,1));
%upleft = candidates_up(left_idx(1),:);
downright = candidates_up(left_idx(1),:);
upright = candidates_up(left_idx(2),:);

[~,left_idx] = sort(candidates_down(:,1));
downleft = candidates_down(left_idx(1),:);
%downright = candidates_down(left_idx(2),:);
upleft = candidates_down(left_idx(2),:);

valid = 0;

if upleft(1) ~= 0 && upright(1) ~= 0 && downleft(1) ~= 0 && downright(1) ~= 0
    valid = 1;
end

end

== matlab function RobotLocalisation_no_external_mode/Routine/Video Localisation/Apply Overlay and send ==
  data: redMask input boolean; greenMask input boolean; red input uint8; green input uint8; blue input uint8; calib input
function fcn(redMask, greenMask, red, green, blue, calib)
%#codegen


persistent tc
if isempty(tc)
    tc = uint32(0);
    if strcmp(coder.target,'rtw')
        coder.ceval('initUDP');
    end
end

sz = size(redMask);
red1 = coder.nullcopy(zeros(sz,'uint8'));
green1 = coder.nullcopy(zeros(sz,'uint8'));
blue1 = coder.nullcopy(zeros(sz,'uint8'));

for ii = 1:numel(redMask)
    if (redMask(ii))
        red1(ii) = uint8(255);
        green1(ii) = uint8(0);
        blue1(ii) = uint8(0);
    else
        red1(ii) = red(ii);
        green1(ii) = green(ii);
        blue1(ii) = blue(ii);
    end
end
if calib
    for ii = 1:numel(redMask)
        if greenMask(ii)
            green1(ii) = uint8(255);
            blue1(ii) = uint8(0);
        end
    end
end

rt = coder.nullcopy(zeros(161,240,'uint8'));
gt = coder.nullcopy(zeros(161,240,'uint8'));
bt = coder.nullcopy(zeros(161,240,'uint8'));

% Write out header frame
rt(1,:) = insertHeader(uint32(1), uint32(tc));
gt(1,:) = insertHeader(uint32(3), uint32(tc));
bt(1,:) = insertHeader(uint32(5), uint32(tc));

% Insert image using a 4 bit colourspace
rt(2:end,:) = bitshift(red1(1:160,:),-4) + bitshift(bitshift(red1(161:320,:),-4),4);
gt(2:end,:) = bitshift(green1(1:160,:),-4) + bitshift(bitshift(green1(161:320,:),-4),4);
bt(2:end,:) = bitshift(blue1(1:160,:),-4) + bitshift(bitshift(blue1(161:320,:),-4),4);


% Send via C
if strcmp(coder.target,'rtw')
    coder.ceval('sendUDP',coder.rref(rt),int32(numel(rt)));
    coder.ceval('sendUDP',coder.rref(gt),int32(numel(gt)));
    coder.ceval('sendUDP',coder.rref(bt),int32(numel(bt)));
end


tc = tc + uint32(1);



function hd = insertHeader(idx, tc)

hd = coder.nullcopy(zeros(1,240,'uint8'));
hd(1,1:4) = typecast(idx,'uint8');
hd(1,5:8) = typecast(tc,'uint8');
hd(1,9:240) = repmat(uint8(255),1,232);

== matlab function RobotLocalisation_no_external_mode/Routine/Video Localisation/Localisation/Get Largest round Blob ==
  data: Area input; id output; Eccentricity input
function id = getMax(Area,Eccentricity)
% getMax  Returns index of the centroid of the largest round blob

%#eml
% E = transpose(Eccentricity);
% Einv = 1./(E+1);
% A = double(transpose(Area));
% criteria = A.*Einv;
% [~, id] = max(criteria);

best_area = int32(0);
id = 1;
for l=1:length(Area)
    if Area(l) > best_area
        if Eccentricity(l) < 0.7
            best_area = Area(l);
            id = l;
        end
    end
end

== matlab function RobotLocalisation_no_external_mode/Routine/Video Localisation/Localisation/Matrix Row Selector ==
  data: id input; in input; out output
function out = selector_mat(id, in)
% getMax  Returns index of the centroid of the largest blob

%#eml
out = in(id,:);

== matlab function RobotLocalisation_no_external_mode/Routine/Video Localisation/Localisation/Matrix element Selector ==
  data: id input; in input; out output
function out = selector(id, in)
% getMax  Returns index of the centroid of the largest blob

%#eml
out = in(id);

== matlab function RobotLocalisation_no_external_mode/Routine/Process input updates ==
  data: data input; size input; ical data_store_memory
function fcn(data,size)
%#codegen

global ical

if size == uint16(176)
    for l=1:22
        sp = 1 + (l-1)*8;
        ical(l) = typecast(data(sp:sp+7),'double');
    end
end

== matlab function RobotLocalisation_no_external_mode/toc ==
  data: u input; y output; u2 input
function y = fcn(u,u2)
%#codegen

tr = double(u(1));
tr1 = tr;

if strcmp(coder.target,'rtw')
    coder.ceval('toc',coder.wref(tr),int32(0));
    coder.ceval('toc',coder.wref(tr1),int32(1));
    coder.ceval('tic',int32(1));
end

y = [typecast([tr tr1 u2],'uint8')];

== matlab function RobotLocalisation_no_external_mode/tic ==
  data: y output
function y = fcn()
%#codegen

if strcmp(coder.target,'rtw')
    coder.ceval('tic',int32(0));
end

y = zeros(1,8,'uint8');

== matlab function RobotLocalisation_no_external_mode/Trigger at 0.2 ==
  events: do output FUNCTION_CALL_EVENT
function fcn
%#codegen

persistent exec
if isempty(exec)
    exec = uint8(0);
end

exec = exec + 1;
if exec >= uint8(5)
    do;
    exec = uint8(0);
end
